simulink model "Forces_estimation"  (R2015a)
settings: Solver=ode2  StartTime=0.0  StopTime=10.0  FixedStep=0.01  RelTol=1e-3
InitFcn:
  | TiltCopter_Parameters_TOSTO_v3
undefined symbols (not defined in the file): degtorad, Kt, x1
settings Model: Creator=pela  LastModifiedBy=Claudio
settings HardwareCC: ProdLargestAtomicInteger=Long  ProdLargestAtomicFloat=Double  ProdEndianess=LittleEndian  ProdHWDeviceType=ARM Compatible->ARM Cortex
settings RTWCC: GenCodeOnly=on  GenerateReport=on  Toolchain=Microsoft Visual C++ 2013 v12.0 | nmake (64-bit Windows)  BuildConfiguration=Faster Runs  LaunchReport=on  TargetLang=C++
settings GRTTargetCC: MatFileLogging=off  MultiInstanceERTCode=on  CodeInterfacePackaging=C++ class

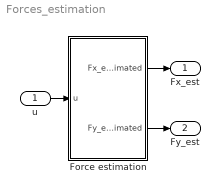
== system Forces_estimation ==
  u : Inport
  Force estimation : Subsystem
  Fx_est : Outport
  Fy_est : Outport  Port=2
  wires:
  u/1 -> Force estimation/1(u)
  Force estimation/1(Fx_estimated) -> Fx_est/1
  Force estimation/2(Fy_estimated) -> Fy_est/1

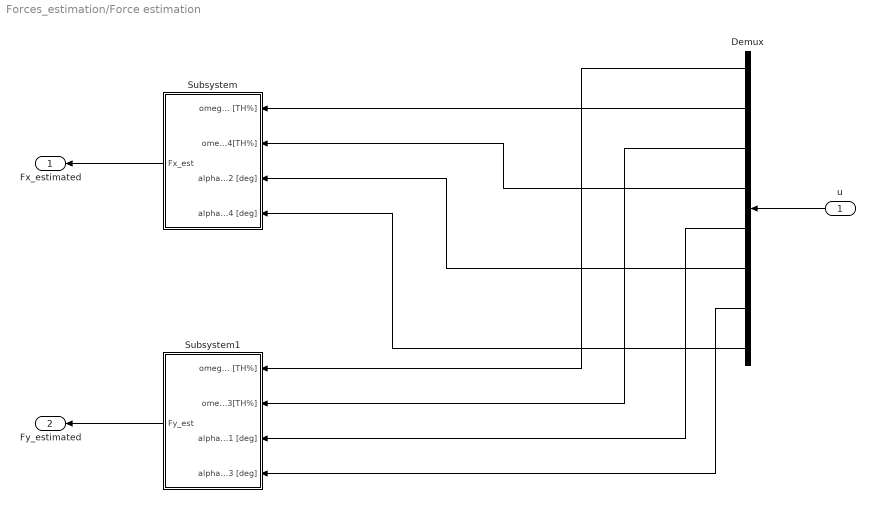
== system Forces_estimation/Force estimation ==
  u : Inport
  Demux : Demux  Outputs=8
  Subsystem : Subsystem
  Subsystem1 : Subsystem
  Fx_estimated : Outport
  Fy_estimated : Outport  Port=2
  wires:
  u/1 -> Demux/1
  Subsystem/1(Fx_est) -> Fx_estimated/1
  Demux/2 -> Subsystem/1(omega_2 [TH%])
  Demux/4 -> Subsystem/2(omega_4[TH%])
  Demux/6 -> Subsystem/3(alpha_2 [deg])
  Demux/8 -> Subsystem/4(alpha_4 [deg])
  Subsystem1/1(Fy_est) -> Fy_estimated/1
  Demux/1 -> Subsystem1/1(omega_1 [TH%])
  Demux/3 -> Subsystem1/2(omega_3[TH%])
  Demux/5 -> Subsystem1/3(alpha_1 [deg])
  Demux/7 -> Subsystem1/4(alpha_3 [deg])

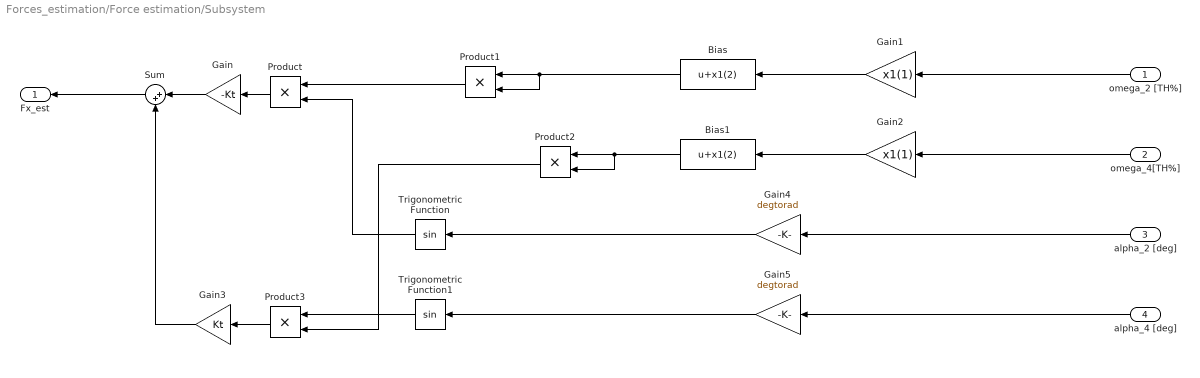
== system Forces_estimation/Force estimation/Subsystem ==
  omega_2 [TH%] : Inport
  omega_4[TH%] : Inport  Port=2
  alpha_2 [deg] : Inport  Port=3
  alpha_4 [deg] : Inport  Port=4
  Bias : Bias  Bias=x1(2)
  Bias1 : Bias  Bias=x1(2)
  Gain : Gain  Gain=-Kt
  Gain1 : Gain  Gain=x1(1)
  Gain2 : Gain  Gain=x1(1)
  Gain3 : Gain  Gain=Kt
  Gain4 : Gain  Gain=degtorad
  Gain5 : Gain  Gain=degtorad
  Product{,1..3} (4 alike) : Product
  Sum : Sum  Inputs=|++
  Trigonometric Function : Trigonometry
  Trigonometric Function1 : Trigonometry
  Fx_est : Outport
  wires:
  Gain3/1 -> Sum/2
  Gain2/1 -> Bias1/1
  omega_4[TH%]/1 -> Gain2/1
  Bias1/1 -> Product2/1, Product2/2
  Gain1/1 -> Bias/1
  Trigonometric Function/1 -> Product/2
  alpha_4 [deg]/1 -> Gain5/1
  Product/1 -> Gain/1
  alpha_2 [deg]/1 -> Gain4/1
  Sum/1 -> Fx_est/1
  omega_2 [TH%]/1 -> Gain1/1
  Product2/1 -> Product3/2
  Gain/1 -> Sum/1
  Bias/1 -> Product1/2, Product1/1
  Trigonometric Function1/1 -> Product3/1
  Product3/1 -> Gain3/1
  Product1/1 -> Product/1
  Gain4/1 -> Trigonometric Function/1
  Gain5/1 -> Trigonometric Function1/1

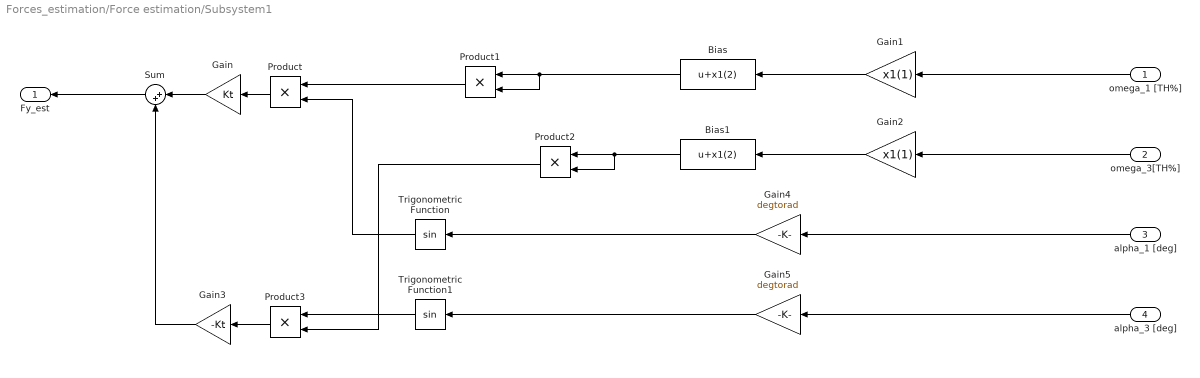
== system Forces_estimation/Force estimation/Subsystem1 ==
  omega_1 [TH%] : Inport
  omega_3[TH%] : Inport  Port=2
  alpha_1 [deg] : Inport  Port=3
  alpha_3 [deg] : Inport  Port=4
  Bias : Bias  Bias=x1(2)
  Bias1 : Bias  Bias=x1(2)
  Gain : Gain  Gain=Kt
  Gain1 : Gain  Gain=x1(1)
  Gain2 : Gain  Gain=x1(1)
  Gain3 : Gain  Gain=-Kt
  Gain4 : Gain  Gain=degtorad
  Gain5 : Gain  Gain=degtorad
  Product{,1..3} (4 alike) : Product
  Sum : Sum  Inputs=|++
  Trigonometric Function : Trigonometry
  Trigonometric Function1 : Trigonometry
  Fy_est : Outport
  wires:
  Gain5/1 -> Trigonometric Function1/1
  Gain4/1 -> Trigonometric Function/1
  Product1/1 -> Product/1
  Product3/1 -> Gain3/1
  Trigonometric Function1/1 -> Product3/1
  Bias/1 -> Product1/1, Product1/2
  Gain/1 -> Sum/1
  Product2/1 -> Product3/2
  omega_1 [TH%]/1 -> Gain1/1
  Sum/1 -> Fy_est/1
  alpha_1 [deg]/1 -> Gain4/1
  Product/1 -> Gain/1
  alpha_3 [deg]/1 -> Gain5/1
  Trigonometric Function/1 -> Product/2
  Gain1/1 -> Bias/1
  Bias1/1 -> Product2/2, Product2/1
  omega_3[TH%]/1 -> Gain2/1
  Gain2/1 -> Bias1/1
  Gain3/1 -> Sum/2
